simulink model "req10"  (R2019a)
settings: Solver=FixedStepAuto  StartTime=0.0  StopTime=100  RelTol=1e-3
settings Model: Creator=e40014285  LastModifiedBy=e40014285
settings ConfigComp: CovEnable=on  RecordCoverage=on  CovHTMLOptions=-sRT=1 -sVT=0 -aTS=1 -bRG=1 -bTC=1 -hTR=0 -nFC=0 -nFD=1 -scm=1 -bcm=1 -xEv=0 -xEM=0  CovHtmlReporting=on  CovCumulativeReport=on  CovModelRefEnable=on  DVModelCoverageObjectives=MCDC  DVTestSuiteOptimization=Auto  DVDetectOutOfBounds=on  DVReportPDFFormat=on  DVRebuildModelRepresentation=Always

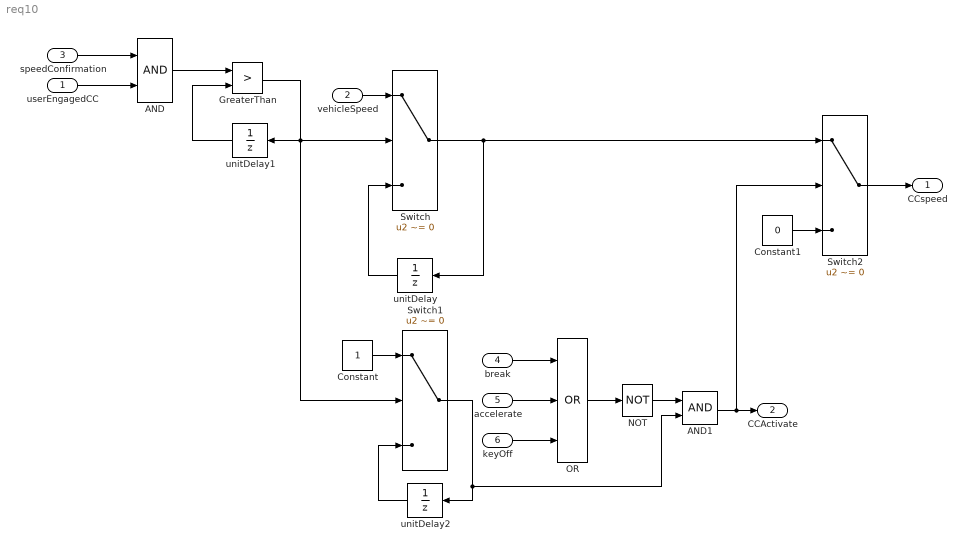
== system req10 ==
  userEngagedCC : Inport
  vehicleSpeed : Inport  Port=2
  speedConfirmation : Inport  Port=3
  break : Inport  Port=4
  accelerate : Inport  Port=5
  keyOff : Inport  Port=6
  AND : Logic  AllPortsSameDT=off  OutDataTypeStr=boolean
  AND1 : Logic  AllPortsSameDT=off  OutDataTypeStr=boolean
  Constant : Constant
  Constant1 : Constant  Value=0
  GreaterThan : RelationalOperator  Operator=>  OutDataTypeStr=boolean  RndMeth=Simplest
  NOT : Logic  Operator=NOT  AllPortsSameDT=off  OutDataTypeStr=boolean
  OR : Logic  Operator=OR  Inputs=3  AllPortsSameDT=off  OutDataTypeStr=boolean
  Switch : Switch  Criteria=u2 ~= 0
  Switch1 : Switch  Criteria=u2 ~= 0
  Switch2 : Switch  Criteria=u2 ~= 0
  unitDelay : UnitDelay  SampleTime=-1  HasFrameUpgradeWarning=on
      settings: AttributesFormatString=InitialValue = %<InitialCondition>
  unitDelay1 : UnitDelay  SampleTime=-1  HasFrameUpgradeWarning=on
      settings: AttributesFormatString=InitialValue = %<InitialCondition>
  unitDelay2 : UnitDelay  SampleTime=-1  HasFrameUpgradeWarning=on
      settings: AttributesFormatString=InitialValue = %<InitialCondition>
  CCspeed : Outport
  CCActivate : Outport  Port=2
  wires:
  speedConfirmation/1 -> AND/1
  vehicleSpeed/1 -> Switch/1
  Switch/1 -> Switch2/1, unitDelay/1
  unitDelay/1 -> Switch/3
  GreaterThan/1 -> Switch1/2, unitDelay1/1, Switch/2
  unitDelay1/1 -> GreaterThan/2
  userEngagedCC/1 -> AND/2
  AND/1 -> GreaterThan/1
  Switch1/1 -> unitDelay2/1, AND1/2
  unitDelay2/1 -> Switch1/3
  Constant/1 -> Switch1/1
  Switch2/1 -> CCspeed/1
  Constant1/1 -> Switch2/3
  break/1 -> OR/1
  accelerate/1 -> OR/2
  keyOff/1 -> OR/3
  OR/1 -> NOT/1
  NOT/1 -> AND1/1
  AND1/1 -> CCActivate/1, Switch2/2
